simulink model "LUTdepth_cost_c"  (Simulink 6.6)
settings: Solver=VariableStepDiscrete  SolverMode=SingleTasking  StartTime=0.0  StopTime=128/100e3  RelTol=1e-3
libraries: xbsIndex_r4 x8
settings Model: Creator=lcrockett  LastModifiedBy=lcrockett
settings DataIOCC: SignalLoggingName=sigsOut
settings DebuggingCC: SignalResolutionControl=TryResolveAllWithWarning  SolverPrmCheckMsg=none  MultiTaskDSMMsg=warning  MultiTaskCondExecSysMsg=none  StrictBusMsg=None
settings HardwareCC: TargetUnknown=on
settings RTWCC: IncludeERTFirstTime=on
settings GRTTargetCC: ModelReferenceCompliant=off  MatFileLogging=off

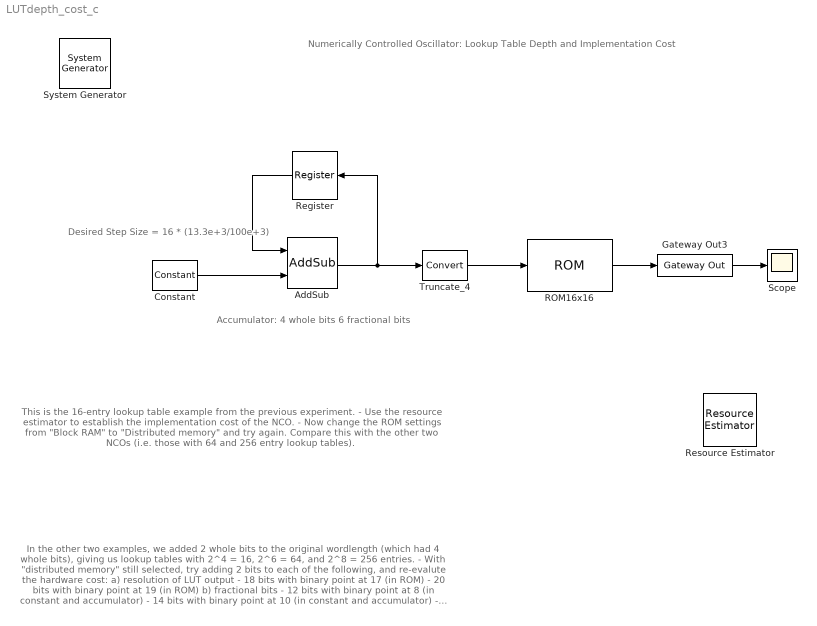
== system LUTdepth_cost_c ==
  note: Numerically Controlled Oscillator:
      | Lookup Table Depth and Implementation Cost
  note: Desired Step Size =
      | 16 * (13.3e+3/100e+3)
  note: Accumulator:
      | 4 whole bits
      | 6 fractional bits
  note: This is the 16-entry lookup table example from the previous experiment.
      | - Use the resource estimator to establish the implementation cost of the NCO.
      | - Now change the ROM settings from "Block RAM" to "Distributed memory"
      |   and try again. Compare this with the other two NCOs (i.e. those with 64 and 256
      |   entry lookup tables).
  note: In the other two examples, we added 2 whole bits to the original wordlength
      | (which had 4 whole bits), giving us lookup tables with 2^4 = 16, 2^6 = 64, and
      | 2^8 = 256 entries.
      | - With "distributed memory" still selected, try adding 2 bits to each of the following,
      |   and re-evalute the hardware cost:
      |     a) resolution of LUT output
      |         - 18 bits with binary point at 17 (in ROM)
      |         - 20 bits with binary point at 19 (in ROM)
      |     b) fractional bits
      |         - 12 bits with binary point at 8 (in constant and accumulator)
      |         - 14 bits with binary point at 10 (in constant and accumulator)
      | - Which parameter (of the three considered here) has the biggest impact on
      |   implementation cost?
  " System Generator" : xbsIndex_r4/ System Generator  Tag=genX  SystemSampleTime=-1  xilinxfamily=virtex2  part=xc2v40  speed=-4  package=cs144  synthesis_tool=XST  clock_wrapper=Clock Enables  directory=./netlist  testbench=off  simulink_period=1/100e3  sysclk_period=50  dcm_input_clock_period=100  incr_netlist=off  trim_vbits=Everywhere in SubSystem  dbl_ovrd=No Where in SubSystem  core_generation=According to Block Masks  run_coregen=off  deprecated_control=off  eval_field=0  block_type=sysgen
      settings: block_version=9.1.01
  AddSub : xbsIndex_r4/AddSub  mode=Addition  use_carryin=off  use_carryout=off  en=off  latency=0  precision=User Defined  arith_type=Unsigned  n_bits=10  bin_pt=6  quantization=Truncate  overflow=Wrap  dbl_ovrd=off  use_behavioral_HDL=on  pipelined=off  use_rpm=on  block_type=addsub
      settings: xl_area=[5 0 0 10 0 0 0]  block_version=VER_STRING_GOES_HERE
  Constant : xbsIndex_r4/Constant  arith_type=Unsigned  const=16*(13.3e+3/100e+3)  n_bits=10  bin_pt=6  explicit_period=on  period=1/100e3  equ=P=C  opselect=C  inp2=PCIN>>17  opr=+  inp1=P  carry=CIN  dbl_ovrd=off  block_type=constant
      settings: block_version=VER_STRING_GOES_HERE
  Gateway Out3 : xbsIndex_r4/Gateway Out  hdl_port=on  timing_constraint=None  locs_specified=off  LOCs={}  block_type=gatewayout
      settings: infoedit="Gateway out block.  Converts Xilinx fixed point inputs into ouputs of type Simulink integer, double, or fixed point.<P><P>Hardware notes:  In hardware these blocks become top level output ports or are discarded, depending on how they are configured."  xl_area=[0 0 0 0 16 0 0]  block_version=VER_STRING_GOES_HERE
  ROM16x16 : xbsIndex_r4/ROM  depth=16  initVector=sin(pi*(0:15)/8)  distributed_mem=Block RAM  rst=off  init_reg=0  en=off  latency=1  arith_type="Signed  (2's comp)"  n_bits=16  bin_pt=15  dbl_ovrd=off  optimize=Area  use_rpm=off  block_type=sprom
      settings: xl_area=[8 16 0 16 0 0 0]  block_version=VER_STRING_GOES_HERE
  Register : xbsIndex_r4/Register  Orientation=left  init=0  rst=off  en=off  dbl_ovrd=off  block_type=register
      settings: xl_area=[5 10 0 0 0 0 0]  block_version=VER_STRING_GOES_HERE
  Resource Estimator : xbsIndex_r4/Resource Estimator  Tag=resEstTag  Slices=0  FFs=0  BRAMs=0  LUTs=0  IOBs=0  EBMs=0  TBUFs=0  xl_use_estimator_area=off  est_options=Estimate  xl_estimator_area=[20 26 0 30 16 0 0]  block_type=resource_estimator
      settings: AttributesFormatString=Resource\nEstimator  block_version=9.1.01
  Scope : Scope
  Truncate_4 : xbsIndex_r4/Convert  arith_type=Unsigned  n_bits=4  bin_pt=0  quantization="Round  (unbiased: +/- Inf)"  overflow=Wrap  latency=0  dbl_ovrd=off  pipeline=off  block_type=convert
      settings: xl_area=[2 0 0 4 0 0 0]  block_version=VER_STRING_GOES_HERE
  wires:
  Constant/1 -> AddSub/2
  AddSub/1 -> Register/1, Truncate_4/1
  Register/1 -> AddSub/1
  Truncate_4/1 -> ROM16x16/1
  ROM16x16/1 -> Gateway Out3/1
  Gateway Out3/1 -> Scope/1
